simulink model "balanceCar2"  (R2023b)
settings: Solver=VariableStepAuto  StartTime=0.0  StopTime=10.0  RelTol=1e-3
settings Model: Creator=xjtu  LastModifiedBy=xjtu

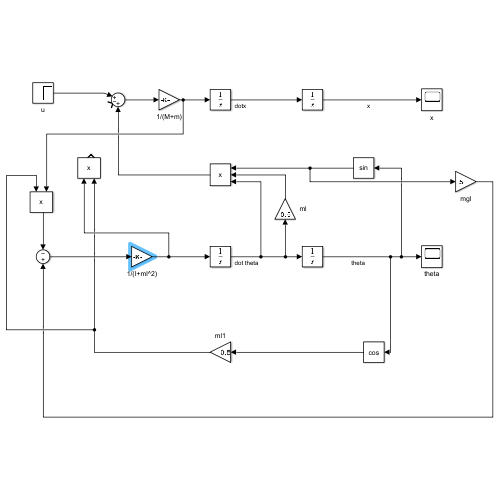
[thumbnail: Simulink's stored preview of the top-level diagram]
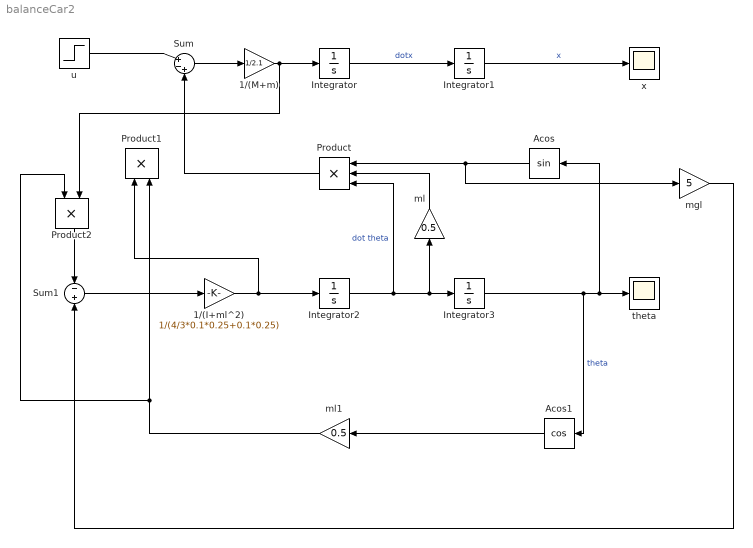
== system balanceCar2 ==
  1/(I+ml^2) : Gain  Gain=1/(4/3*0.1*0.25+0.1*0.25)
  1/(M+m) : Gain  Gain=1/2.1
  Acos : Trigonometry
  Acos1 : Trigonometry  Operator=cos
  Integrator : Integrator
  Integrator1 : Integrator
  Integrator2 : Integrator
  Integrator3 : Integrator  InitialCondition=pi/6
  Product : Product  Inputs=3
  Product1 : Product
  Product2 : Product
  Sum : Sum  Inputs=|+-+
  Sum1 : Sum  Inputs=-|+
  mgl : Gain  Gain=5
  ml : Gain  Gain=0.5
  ml1 : Gain  Gain=0.5
  theta : Scope
  u : Step  Time=0  After=0  SampleTime=0
  x : Scope
  wires:
  Integrator2/1 -> Product/3, Integrator3/1, ml/1  "dot theta"
  Integrator3/1 -> Acos1/1, Acos/1, theta/1  "theta"
  Integrator1/1 -> x/1  "x"
  Integrator/1 -> Integrator1/1  "dotx"
  u/1 -> Sum/1
  1/(M+m)/1 -> Integrator/1, Product2/2
  Sum/1 -> 1/(M+m)/1
  Sum1/1 -> 1/(I+ml^2)/1
  Acos/1 -> mgl/1, Product/1
  ml/1 -> Product/2
  Product/1 -> Sum/3
  ml1/1 -> Product2/1, Product1/2
  Acos1/1 -> ml1/1
  1/(I+ml^2)/1 -> Integrator2/1, Product1/1
  mgl/1 -> Sum1/2
  Product2/1 -> Sum1/1
